simulink model "main"  (Simulink 3.00)
libraries: genlib x2, speclib x1, matrixlib x1, arclib x1

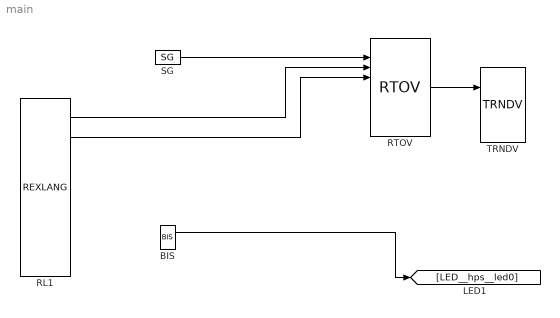
== system main ==
  BIS : genlib/BIS  Y0=off  t1=0.2  t2=0.4  t3=0.0000000E+000  t4=4.0000000E+000  t5=5.0000000E+000  t6=6.0000000E+000  t7=7.0000000E+000  t8=8.0000000E+000  RPT=on
  RL1 : speclib/REXLANG  srcname=rl1.stl  srctype=1: STL  debug=1: No check  fname=datafile.dat  stack=0  strs=0  p0=0x638
  RTOV : matrixlib/RTOV  capacity=8  offset=0  n=8  Type=8: Double
  SG : genlib/SG  isig=1: SINE  amp=1.0000000E+000  freq=1.0000000E+000  phase=0.0000000E+000  ifrunit=1: Hz  iphunit=1: degrees
  TRNDV : arclib/TRNDV  n=8  l=1000  btype=8: Double  pfac=1  afac=0  arc=0  id=1  Title=Trend Title
  wires:
  BIS/1 -> [LED__hps__led0]
  RL1/2 -> RTOV/3
  RL1/4 -> RTOV/4
  RTOV/1 -> TRNDV/1
  SG/1 -> RTOV/2
